simulink model "s10_challenge_simul"  (R2022b)
settings: Solver=FixedStepAuto  StartTime=0.0  StopTime=10  FixedStep=0.001  RelTol=1e-3
values from neighbouring files (symbols this model uses):
  challenge =     [challenge.mat]
undefined symbols (not defined in the file or in its folder): DiscIntNeverNeededParam, National_Instruments, PCI, sens, simul, Ts
libraries: sldrtlib x3
settings Model: SimulationMode=external  ExtModeTrigDuration=1000001  ExtModeTrigDurationFloating=50001  Creator=perondavid  LastModifiedBy=perondavid
settings DataIOCC: LoggingToFile=on
settings HardwareCC: ProdBitPerLong=64  ProdHWDeviceType=Intel->x86-64 (Linux 64)
settings RTWCC: Description=Simulink Desktop Real-Time  SystemTargetFile=sldrt.tlc  TemplateMakefile=sldrt.tmf  RTWCompilerOptimization=on
settings CodeAppCC: MaxIdLength=95
settings SimulinkDesktopRealTimeCC: TargetLibSuffix=_sldrt.a  TargetPreCompLibLocation=C:\Program Files\MATLAB\R2022b\toolbox\sldrt\lib\win64

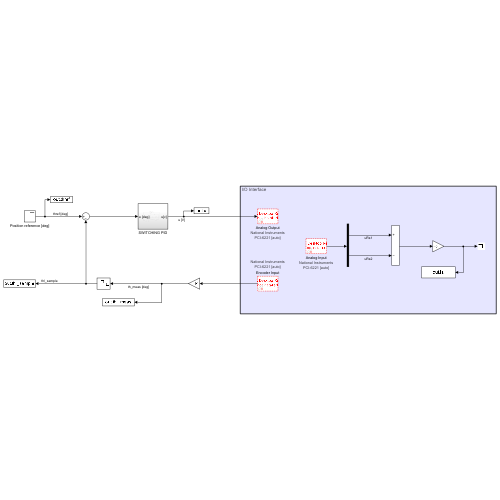
[thumbnail: Simulink's stored preview of the top-level diagram]
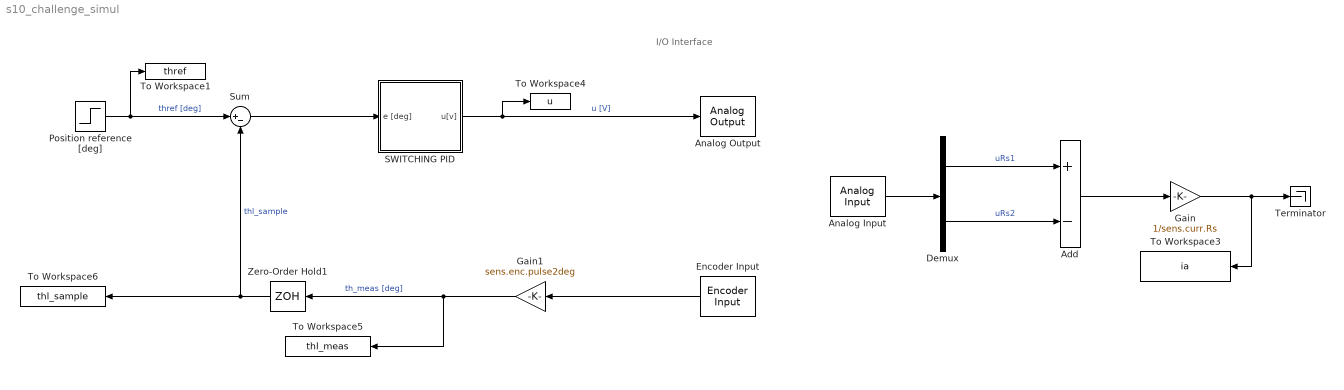
== system s10_challenge_simul ==
  note: I/O Interface
  Add : Sum  Inputs=+-
  Analog Input : sldrtlib/Analog Input  SampleTime=-1  MaxMissedTicks=10  ShowMissedTicks=off  YieldWhenWaiting=off  DrvName=National_Instruments/PCI-6221  DrvAddress=4294967295  DrvOptions=[0 0 0 2 0]  Channels=[1, 2]  RangeMode=1  VoltRange=1  DataType=1
      settings: AttributesFormatString=National Instruments\nPCI-6221 [auto]
  Analog Output : sldrtlib/Analog Output  SampleTime=-1  MaxMissedTicks=10  ShowMissedTicks=off  YieldWhenWaiting=off  DrvName=National_Instruments/PCI-6221  DrvAddress=4294967295  DrvOptions=[0 0 0 2 0]  Channels=1  RangeMode=1  VoltRange=1  InitialValue=0  FinalValue=0
      settings: AttributesFormatString=National Instruments\nPCI-6221 [auto]
  Demux : Demux  Outputs=2
  Encoder Input : sldrtlib/Encoder Input  SampleTime=-1  MaxMissedTicks=10  ShowMissedTicks=off  YieldWhenWaiting=off  DrvName=National_Instruments/PCI-6221  DrvAddress=4294967295  DrvOptions=[0 0 0 2 0]  Channels=1  QuadMode=3  IndexPulse=1  InputFilter=Inf  DataType=1
      settings: AttributesFormatString=National Instruments\nPCI-6221 [auto]
  Gain : Gain  Gain=1/sens.curr.Rs
  Gain1 : Gain  Gain=sens.enc.pulse2deg
  Position reference [deg] : Step  Time=0  After=simul.stepdeg  SampleTime=challenge.Ts
  SWITCHING PID : Subsystem
  Sum : Sum  Inputs=|+-
  Terminator : Terminator
  To Workspace1 : ToWorkspace  VariableName=thref  SaveFormat=Structure With Time  SampleTime=Ts
  To Workspace3 : ToWorkspace  VariableName=ia  SaveFormat=Structure With Time  SampleTime=Ts
  To Workspace4 : ToWorkspace  VariableName=u  SaveFormat=Structure With Time  SampleTime=Ts
  To Workspace5 : ToWorkspace  VariableName=thl_meas  SaveFormat=Structure With Time  SampleTime=Ts
  To Workspace6 : ToWorkspace  VariableName=thl_sample  SaveFormat=Structure With Time  SampleTime=Ts
  Zero-Order Hold1 : ZeroOrderHold  SampleTime=challenge.Ts
  wires:
  Demux/1 -> Add/1  "uRs1"
  Demux/2 -> Add/2  "uRs2"
  Add/1 -> Gain/1
  Gain/1 -> To Workspace3/1, Terminator/1
  Analog Input/1 -> Demux/1
  SWITCHING PID/1(u[v]) -> Analog Output/1, To Workspace4/1  "u [V]"
  Gain1/1 -> To Workspace5/1, Zero-Order Hold1/1  "th_meas [deg]"
  Sum/1 -> SWITCHING PID/1(e [deg])
  Position reference [deg]/1 -> Sum/1, To Workspace1/1  "thref [deg]"
  Zero-Order Hold1/1 -> To Workspace6/1, Sum/2  "thl_sample"
  Encoder Input/1 -> Gain1/1

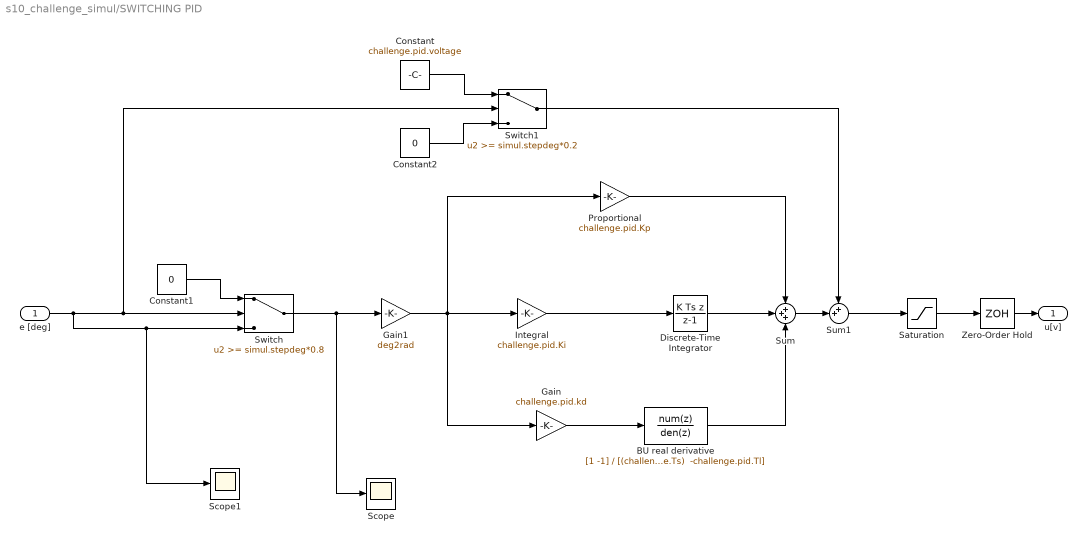
== system s10_challenge_simul/SWITCHING PID ==
  e [deg] : Inport
  BU real derivative : DiscreteTransferFcn  Numerator=[1 -1]  Denominator="[(challenge.pid.Tl+challenge.Ts)  -challenge.pid.Tl]"  SampleTime=challenge.Ts
  Constant : Constant  Value=challenge.pid.voltage
  Constant1 : Constant  Value=0
  Constant2 : Constant  Value=0
  Discrete-Time Integrator : DiscreteIntegrator  IntegratorMethod=Integration: Backward Euler  SampleTime=challenge.Ts  ICPrevOutput=DiscIntNeverNeededParam  ICPrevScaledInput=DiscIntNeverNeededParam
  Gain : Gain  Gain=challenge.pid.kd
  Gain1 : Gain  Gain=deg2rad
  Integral : Gain  Gain=challenge.pid.Ki
  Proportional : Gain  Gain=challenge.pid.Kp
  Saturation : Saturate  UpperLimit=10  LowerLimit=-10
  Scope : Scope
  Scope1 : Scope
  Sum : Sum  Inputs=+++
  Sum1 : Sum  Inputs=++|
  Switch : Switch  Threshold=simul.stepdeg*0.8  SaturateOnIntegerOverflow=off  InputSameDT=off
  Switch1 : Switch  Threshold=simul.stepdeg*0.2  SaturateOnIntegerOverflow=off  InputSameDT=off
  Zero-Order Hold : ZeroOrderHold  SampleTime=challenge.Ts
  u[v] : Outport
  wires:
  e [deg]/1 -> Scope1/1, Switch/3, Switch/2, Switch1/2
  Zero-Order Hold/1 -> u[v]/1
  Saturation/1 -> Zero-Order Hold/1
  Proportional/1 -> Sum/1
  Integral/1 -> Discrete-Time Integrator/1
  Discrete-Time Integrator/1 -> Sum/2
  BU real derivative/1 -> Sum/3
  Gain/1 -> BU real derivative/1
  Gain1/1 -> Proportional/1, Gain/1, Integral/1
  Constant/1 -> Switch1/1
  Switch/1 -> Scope/1, Gain1/1
  Constant1/1 -> Switch/1
  Constant2/1 -> Switch1/3
  Sum1/1 -> Saturation/1
  Sum/1 -> Sum1/2
  Switch1/1 -> Sum1/1
